simulink model "Diagrama_de_Blocos"  (R2018b)
settings: Solver=FixedStepAuto  StartTime=0.0  StopTime=300  FixedStep=1e-3  RelTol=1e-3
undefined symbols (not defined in the file): A, du1, hb, k1, k2, u1b, u2
settings Model: Creator=davi2  LastModifiedBy=davi2
settings DataIOCC: SaveOutput=off  SignalLogging=off  DSMLogging=off  TimeSaveName=t

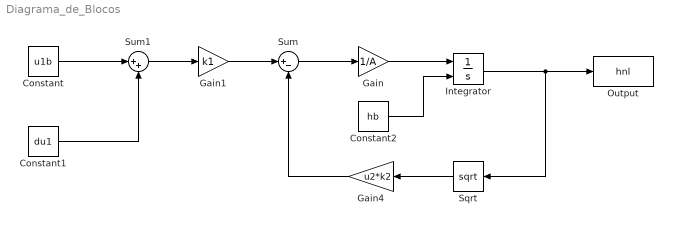
== system Diagrama_de_Blocos ==
  Constant : Constant  Value=u1b
  Constant1 : Constant  Value=du1
  Constant2 : Constant  Value=hb
  Gain : Gain  Gain=1/A
  Gain1 : Gain  Gain=k1
  Gain4 : Gain  Gain=u2*k2
  Integrator : Integrator  InitialConditionSource=external
  Output : ToWorkspace  VariableName=hnl  SampleTime=-1
  Sqrt : Sqrt  SaturateOnIntegerOverflow=on
  Sum : Sum  Inputs=|+-
  Sum1 : Sum  Inputs=|++
  wires:
  Sqrt/1 -> Gain4/1
  Gain1/1 -> Sum/1
  Sum/1 -> Gain/1
  Gain4/1 -> Sum/2
  Constant/1 -> Sum1/1
  Gain/1 -> Integrator/1
  Integrator/1 -> Output/1, Sqrt/1
  Constant2/1 -> Integrator/2
  Sum1/1 -> Gain1/1
  Constant1/1 -> Sum1/2
